simulink model "exp04p02"  (R2021a)
settings: Solver=VariableStepAuto  StartTime=0.0  StopTime=10.0  RelTol=1e-3
libraries: spsThyristorLib x2, spsVoltageMeasurementLib x2, spsACVoltageSourceLib x1, spsPLLLib x1, spsRMSLib x1, spsSampleandHoldLib x1, spsSeriesRLCBranchLib x1, spspowerguiLib x1
settings Model: Creator=User  LastModifiedBy=User

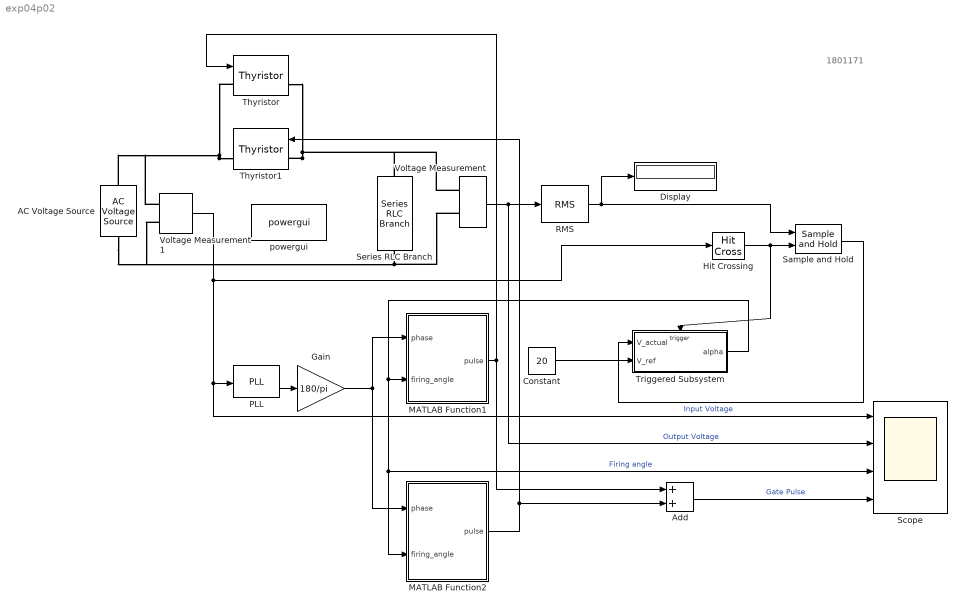
== system exp04p02 ==
  note: 1801171
  AC Voltage Source : spsACVoltageSourceLib/AC Voltage Source  Amplitude=100  Phase=0  Frequency=50  SampleTime=0  Measurements=None  BusType=swing  Pref=10e3  Qref=0  Qmin=-inf  Qmax=+inf
  Add : Sum
  Constant : Constant  Value=20
  Display : Display
  Gain : Gain  Gain=180/pi
  Hit Crossing : HitCross
  MATLAB Function1 : MATLAB Function  TreatAsAtomicUnit=on
  MATLAB Function2 : MATLAB Function  TreatAsAtomicUnit=on
  PLL : spsPLLLib/PLL  Fmin=45  Par_Init=[0, 50]  ParK=[180, 3200, 1]  TcD=1e-4  MaxRateChangeFreq=12  FilterCutOffFreq=25  Ts=0  AGC=on
      settings: SourceProductBaseCode=PS
  RMS : spsRMSLib/RMS  TrueRMS=on  Freq=50  RMSInit=100  Ts=0
  Sample and Hold : spsSampleandHoldLib/Sample and Hold  ic=0  Ts=0
      settings: SourceProductBaseCode=PS
  Scope : Scope  NumInputPorts=4
  Series RLC Branch : spsSeriesRLCBranchLib/Series RLC Branch  LConnTagsString=__new0  RConnTagsString=__new0  BranchType=R  Resistance=10  Inductance=1e-3  SetiL0=off  InitialCurrent=0  Capacitance=1e-6  Setx0=off  InitialVoltage=0  Measurements=None
  Thyristor : spsThyristorLib/Thyristor  Ron=0.001  Lon=0  Vf=0.8  IC=0  Rs=500  Cs=250e-9  Measurements=on
  Thyristor1 : spsThyristorLib/Thyristor  Ron=0.001  Lon=0  Vf=0.8  IC=0  Rs=500  Cs=250e-9  Measurements=on
  Triggered Subsystem : Subsystem  TreatAsAtomicUnit=on
  Voltage Measurement : spsVoltageMeasurementLib/Voltage Measurement  PhasorSimulation=off  OutputType=Complex  PSBequivalent=0
  Voltage Measurement1 : spsVoltageMeasurementLib/Voltage Measurement  PhasorSimulation=off  OutputType=Complex  PSBequivalent=0
  powergui : spspowerguiLib/powergui  Priority=1  SimulationMode=Discrete  SampleTime=50e-6  frequency=60  Iterations=50  frequencyindice=50  Pbase=100e6  ErrMax=1e-4  UnitsV=kV  UnitsW=MW  buscounter=0  FunctionMessages=off  echomessages=off  EnableUseOfTLC=off  CurrentSourceSwitches=off  DisableSnubberDevices=off  DisableRonSwitches=off  DisableVfSwitches=off  DisplayEquations=off  AutomaticDiscreteSolvers=off  SolverType=Tustin/Backward Euler (TBE)  Interpol=off  ExternalGateDelay=off  methode=off  Ts=100  x0status=blocks  SPID=on  SwTol=0  HookPort=off  NonlinearTolerance=1e-4  nMaxIteration=100  ContinueOnMaxIteration=off  RestoreLinks=warning  ResistiveCurrentMeasurement=off  Frange=[0:2:500]  Ylog=off  Xlog=on  ShowGrid=off  save=off  variable=ZData  structure=0  ZoomFFT=off  StartTime=0.0  cycles=1  DisplayStyle=1  fundamental=60  FreqAxis=off  MaxFrequency=1000  frequencyindicesteady=1  RmsSteady=1  display=off
  wires:
  Hit Crossing/1 -> Sample and Hold/2, Triggered Subsystem/Trigger
  Constant/1 -> Triggered Subsystem/2(V_ref)
  Add/1 -> Scope/4  "Gate Pulse"
  Gain/1 -> MATLAB Function2/1(phase), MATLAB Function1/1(phase)
  PLL/2 -> Gain/1
  RMS/1 -> Sample and Hold/1, Display/1
  Sample and Hold/1 -> Triggered Subsystem/1(V_actual)
  Voltage Measurement/1 -> Scope/2, RMS/1  "Output Voltage"
  MATLAB Function2/1(pulse) -> Thyristor1/1, Add/2
  Voltage Measurement1/1 -> Scope/1, PLL/1, Hit Crossing/1  "Input Voltage"
  MATLAB Function1/1(pulse) -> Add/1, Thyristor/1
  Triggered Subsystem/1(alpha) -> Scope/3, MATLAB Function2/2(firing_angle), MATLAB Function1/2(firing_angle)  "Firing angle"
  connections:
  Thyristor1/LConn1 -- Series RLC Branch/LConn1 -- Voltage Measurement/LConn1 -- Thyristor/RConn1
  Series RLC Branch/RConn1 -- AC Voltage Source/LConn1 -- Voltage Measurement1/LConn2 -- Voltage Measurement/LConn2
  Thyristor1/RConn1 -- Voltage Measurement1/LConn1 -- AC Voltage Source/RConn1 -- Thyristor/LConn1

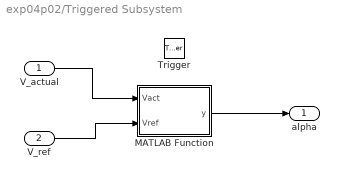
== system exp04p02/Triggered Subsystem ==
  V_actual : Inport
  V_ref : Inport  Port=2
  Trigger : TriggerPort  VariantControl=Variant
  MATLAB Function : MATLAB Function  TreatAsAtomicUnit=on
  alpha : Outport
  wires:
  MATLAB Function/1(y) -> alpha/1
  V_actual/1 -> MATLAB Function/1(Vact)
  V_ref/1 -> MATLAB Function/2(Vref)

== matlab function exp04p02/Triggered Subsystem/MATLAB Function ==
  data: Vact input; y output; Vref input
function y = fcn(Vact,Vref)
step = 1.5;
%code_gen
persistent firing_angle
if isempty(firing_angle), firing_angle=10; end
if Vact<Vref
    firing_angle = firing_angle -step;
    if firing_angle<0 
        firing_angle =0;
    end
elseif Vact>Vref
    firing_angle =firing_angle+step;
    if firing_angle>180
        firing_angle =180;
    end
else 
    firing_angle =firing_angle;
end
y = firing_angle;
end

== matlab function exp04p02/MATLAB Function2 ==
  data: phase input; firing_angle input; pulse output
function pulse = fcn(phase,firing_angle)
pulse_width = 10;

if (phase >=firing_angle+180)&& phase<= min(firing_angle+pulse_width+180,360)
    pulse =1;
else
    pulse=0;
end
end

== matlab function exp04p02/MATLAB Function1 ==
  data: phase input; firing_angle input; pulse output
function pulse = fcn(phase,firing_angle)
pulse_width = 10;

if (phase>=firing_angle)&& phase<= min(firing_angle+pulse_width,180)
    pulse =1;
else
    pulse=0;
end
end
